simulink model "CRC_withLDPC"  (R2022a)
settings: Solver=VariableStepAuto  StartTime=0.0  StopTime=60  RelTol=1e-3
libraries: dspsrcs4 x6, whdledac x2, whdlutilities x1, xilinxrfsoclib x1
settings Model: Creator=Zeyan Wu  LastModifiedBy=endit

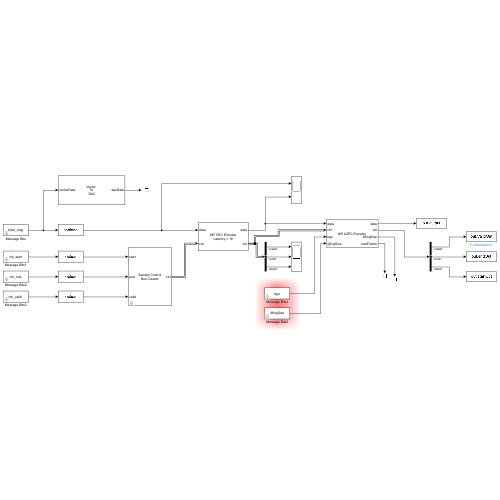
[thumbnail: Simulink's stored preview of the top-level diagram]
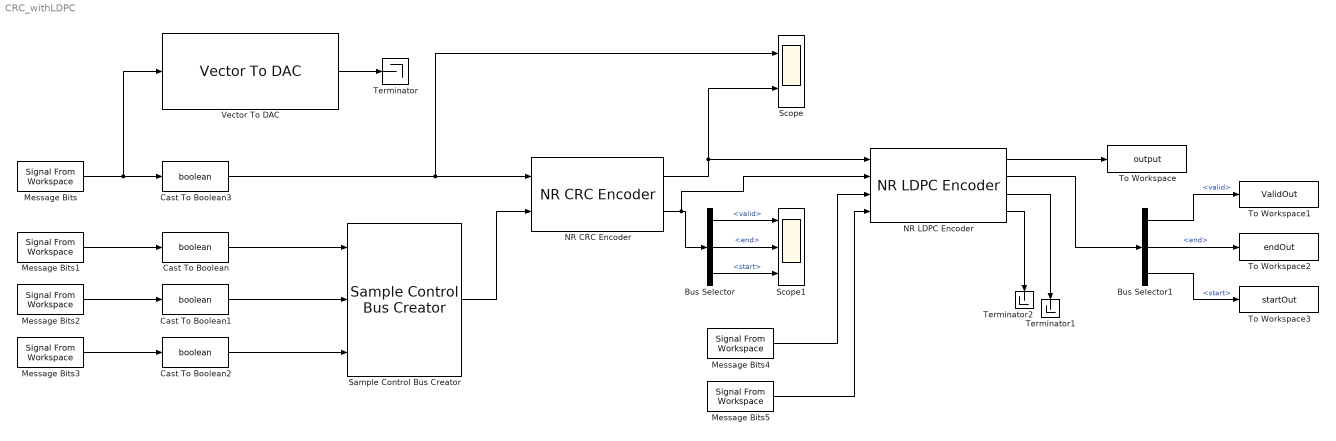
== system CRC_withLDPC ==
  Bus Selector : BusSelector  OutputSignals=valid,end,start
  Bus Selector1 : BusSelector  OutputSignals=valid,end,start
  Cast To Boolean{,1..3} (4 alike) : DataTypeConversion  OutDataTypeStr=boolean  SaturateOnIntegerOverflow=off  RndMeth=Floor
  Message Bits : dspsrcs4/Signal From Workspace  X=input_msg  Ts=1  nsamps=1  OutputAfterFinalValue=Setting to zero  ignoreOrWarnInputAndFrameLengths=off  OutputFrames=on
  Message Bits1 : dspsrcs4/Signal From Workspace  X=ctrl_start  Ts=1  nsamps=1  OutputAfterFinalValue=Setting to zero  ignoreOrWarnInputAndFrameLengths=off  OutputFrames=on
  Message Bits2 : dspsrcs4/Signal From Workspace  X=ctrl_end  Ts=1  nsamps=1  OutputAfterFinalValue=Setting to zero  ignoreOrWarnInputAndFrameLengths=off  OutputFrames=on
  Message Bits3 : dspsrcs4/Signal From Workspace  X=ctrl_valid  Ts=1  nsamps=1  OutputAfterFinalValue=Setting to zero  ignoreOrWarnInputAndFrameLengths=off  OutputFrames=on
  Message Bits4 : dspsrcs4/Signal From Workspace  X=bgn  Ts=1  nsamps=1  OutputAfterFinalValue=Setting to zero  ignoreOrWarnInputAndFrameLengths=off  OutputFrames=on
  Message Bits5 : dspsrcs4/Signal From Workspace  X=liftingSize  Ts=1  nsamps=1  OutputAfterFinalValue=Setting to zero  ignoreOrWarnInputAndFrameLengths=off  OutputFrames=on
  NR CRC Encoder : whdledac/NR CRC Encoder  CRCType=CRC16  EnableCRCMaskPort=off  SimulateUsing=Code generation
      settings: SourceProductBaseCode=LH
  NR LDPC Encoder : whdledac/NR LDPC Encoder
      settings: SourceProductBaseCode=LH
  Sample Control Bus Creator : whdlutilities/Sample Control Bus Creator
      settings: SourceProductBaseCode=LH
  Scope : Scope  NumInputPorts=2
  Scope1 : Scope  NumInputPorts=3
  Terminator : Terminator
  Terminator1 : Terminator
  Terminator2 : Terminator
  To Workspace : ToWorkspace  VariableName=output  SampleTime=1
      settings: Save2DSignal=2-D array (concatenate along first dimension)
  To Workspace1 : ToWorkspace  VariableName=ValidOut  SampleTime=1
      settings: Save2DSignal=2-D array (concatenate along first dimension)
  To Workspace2 : ToWorkspace  VariableName=endOut  SampleTime=1
      settings: Save2DSignal=2-D array (concatenate along first dimension)
  To Workspace3 : ToWorkspace  VariableName=startOut  SampleTime=1
      settings: Save2DSignal=2-D array (concatenate along first dimension)
  Vector To DAC : xilinxrfsoclib/Vector To DAC  INPUT_WL=16  DT_INPUT=0
      settings: SourceProductBaseCode=XILINX_BLOCKSET
  wires:
  Message Bits2/1 -> Cast To Boolean1/1
  Message Bits1/1 -> Cast To Boolean/1
  Message Bits3/1 -> Cast To Boolean2/1
  Sample Control Bus Creator/1 -> NR CRC Encoder/2
  Cast To Boolean/1 -> Sample Control Bus Creator/1
  Cast To Boolean1/1 -> Sample Control Bus Creator/2
  Cast To Boolean2/1 -> Sample Control Bus Creator/3
  NR CRC Encoder/2 -> NR LDPC Encoder/2, Bus Selector/1
  Bus Selector/1 -> Scope1/1  "<valid>"
  Bus Selector/3 -> Scope1/3  "<start>"
  NR CRC Encoder/1 -> NR LDPC Encoder/1, Scope/2
  Bus Selector/2 -> Scope1/2  "<end>"
  Message Bits/1 -> Cast To Boolean3/1, Vector To DAC/1
  Cast To Boolean3/1 -> Scope/1, NR CRC Encoder/1
  Vector To DAC/1 -> Terminator/1
  NR LDPC Encoder/1 -> To Workspace/1
  NR LDPC Encoder/2 -> Bus Selector1/1
  Bus Selector1/1 -> To Workspace1/1  "<valid>"
  Bus Selector1/2 -> To Workspace2/1  "<end>"
  Bus Selector1/3 -> To Workspace3/1  "<start>"
  NR LDPC Encoder/3 -> Terminator1/1
  NR LDPC Encoder/4 -> Terminator2/1
  Message Bits4/1 -> NR LDPC Encoder/3
  Message Bits5/1 -> NR LDPC Encoder/4
